simulink model "KinematicModelG"  (R2016b)
settings: Solver=ode45  StartTime=0.0  StopTime=2  RelTol=1e-3
settings Model: Creator=Daslab  LastModifiedBy=Daslab
settings SolverCC: ShapePreserveControl=EnableAll

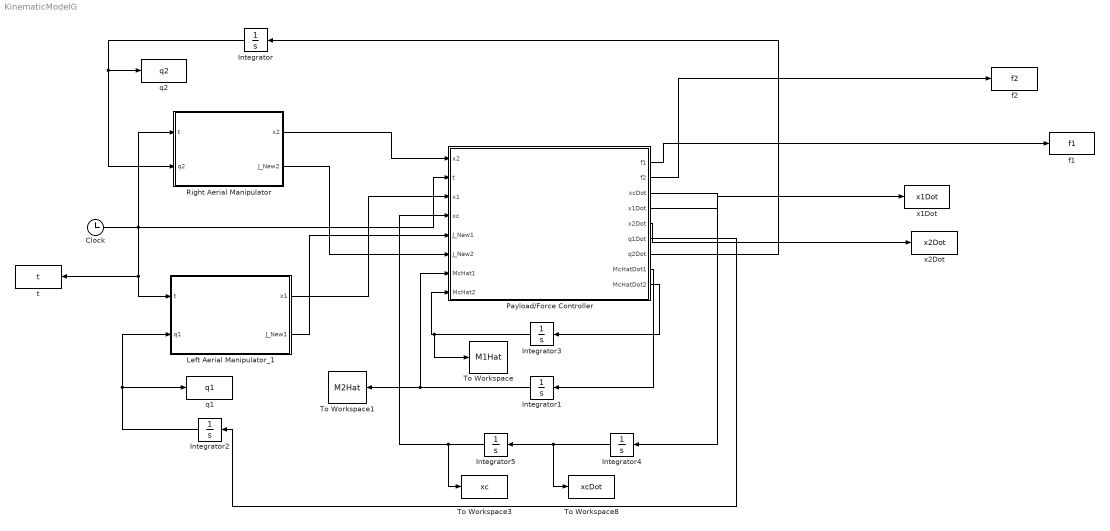
== system KinematicModelG ==
  Clock : Clock
  Integrator : Integrator  InitialCondition=[0.0;0.35;0.68;0;0;0.1;0;pi/2];
  Integrator1 : Integrator
  Integrator2 : Integrator  InitialCondition=[0.1;-0.35;0.7;0;0;-0.1;0;-pi/2];
  Integrator3 : Integrator
  Integrator4 : Integrator  InitialCondition=[0;0;0]
  Integrator5 : Integrator  InitialCondition=[0;0;0.5]
  Left Aerial Manipulator_1 : MATLAB Function  TreatAsAtomicUnit=on
  Payload/Force Controller : MATLAB Function  TreatAsAtomicUnit=on
  Right Aerial Manipulator : MATLAB Function  TreatAsAtomicUnit=on
  To Workspace : ToWorkspace  VariableName=M1Hat  SampleTime=-1
      settings: Save2DSignal=2-D array (concatenate along first dimension)
  To Workspace1 : ToWorkspace  VariableName=M2Hat  SampleTime=-1
      settings: Save2DSignal=2-D array (concatenate along first dimension)
  To Workspace3 : ToWorkspace  VariableName=xc  SampleTime=-1
  To Workspace8 : ToWorkspace  VariableName=xcDot  SampleTime=-1
  f1 : ToWorkspace  VariableName=f1  SampleTime=-1
  "f2 " : ToWorkspace  VariableName=f2  SampleTime=-1
  q1 : ToWorkspace  VariableName=q1  SampleTime=-1
  q2 : ToWorkspace  VariableName=q2  SampleTime=-1
  t : ToWorkspace  VariableName=t  SampleTime=-1
  x1Dot : ToWorkspace  VariableName=x1Dot  SampleTime=-1
  x2Dot : ToWorkspace  VariableName=x2Dot  SampleTime=-1
  wires:
  Integrator/1 -> q2/1, Right Aerial Manipulator/2(q2)
  Clock/1 -> t/1, Left Aerial Manipulator_1/1(t), Right Aerial Manipulator/1(t), Payload/Force Controller/2(t)
  Left Aerial Manipulator_1/1(x1) -> Payload/Force Controller/3(x1)
  Right Aerial Manipulator/1(x2) -> Payload/Force Controller/1(x2)
  Integrator4/1 -> To Workspace8/1, Integrator5/1
  Payload/Force Controller/3(xcDot) -> Integrator4/1
  Integrator5/1 -> To Workspace3/1, Payload/Force Controller/4(xc)
  Payload/Force Controller/1(f1) -> f1/1
  Payload/Force Controller/2(f2) -> "f2 "/1
  Payload/Force Controller/6(q1Dot) -> Integrator2/1
  Integrator2/1 -> q1/1, Left Aerial Manipulator_1/2(q1)
  Payload/Force Controller/5(x2Dot) -> x2Dot/1
  Payload/Force Controller/4(x1Dot) -> x1Dot/1
  Payload/Force Controller/7(q2Dot) -> Integrator/1
  Right Aerial Manipulator/2(J_New2) -> Payload/Force Controller/6(J_New2)
  Left Aerial Manipulator_1/2(J_New1) -> Payload/Force Controller/5(J_New1)
  Payload/Force Controller/9(McHatDot2) -> Integrator3/1
  Integrator3/1 -> To Workspace/1, Payload/Force Controller/8(McHat2)
  Payload/Force Controller/8(McHatDot1) -> Integrator1/1
  Integrator1/1 -> To Workspace1/1, Payload/Force Controller/7(McHat1)

== matlab function KinematicModelG/Left Aerial Manipulator_1 ==
  data: t input; x1 output; q1 input; J_New1 output
function [x1,J_New1] = LeftAerialManipulator(t,q1)
%Kinematics of Left Aerial Manipulator
xb1 = q1(1); 
yb1 = q1(2);
zb1 = q1(3);
psi1 = q1(4);      % z angle in the order ZYX [psi1 theta1 phi1] -->> [Zangle Yangle Xangle]
theta1 = q1(5);    % y angle
phi1 = q1(6);      % x angle 
n11 = q1(7); 
n21 = q1(8);

x_dot1 = 0.2;
y_dot1 = 0.2;
z_dot1 = 0;
phi_dot1 = 0.02;  % x angle 
theta_dot1 = 0;   % y anlge 
psi_dot1 = 0;     % z angle  in the order ZYX  [psiDot thetaDot phiDot] -->> [z y x]Dot
n1_dot1 = 0;
n2_dot1 = 0;

mUAV = 5.0; 
mLink1 = 0.5; 
mLink2 = 0.5;
l1 = 0.2; 
l2 = 0.2;
 
m1 = mUAV + mLink1 + mLink2; 

% Rotation matrix
R_b1 = [ cos(psi1)*cos(theta1), cos(psi1)*sin(phi1)*sin(theta1) - cos(phi1)*sin(psi1), sin(phi1)*sin(psi1) + cos(phi1)*cos(psi1)*sin(theta1); 
      cos(theta1)*sin(psi1), cos(phi1)*cos(psi1) + sin(phi1)*sin(psi1)*sin(theta1),   cos(phi1)*sin(psi1)*sin(theta1) - cos(psi1)*sin(phi1);
      -sin(theta1),         cos(theta1)*sin(phi1),                              cos(phi1)*cos(theta1)];

  
T_b1 = [ 0, -sin(psi1), cos(psi1)*cos(theta1); 
        0,  cos(psi1), cos(theta1)*sin(psi1); 
        1,         0,         -sin(theta1)];

% Forward Kinematics
p_b = [xb1 yb1 zb1]'; %postion of UAV with respect to inertial frame
p_b_dot1 = [x_dot1 y_dot1 z_dot1]';
n_dot1 = [n1_dot1 n2_dot1]'; % joint angles rate 
h1 = [1 0 0]'; 
P10 = [0 0 0.0]';
p1c = [0 0 -l1/2]';

R01 = expm((hat(h1))*n11);

p1c_b = P10 + R01*p1c;    % in base frame 
p1c_i = p_b + R_b1*p1c_b;  % in inertial frame

% position of center of link 2 
h2 = [0 1 0]';
p12 = [0 0 -l1]';
p2T = [0 l2 0]';
p2c = [0 l2/2 0]';

R12 = expm((hat(h2))*n21);
R02 = R01*R12;

% position of end effector 
p2_b1 = P10 + R01*p12 + R02*p2T; % in base frame
% disp(p2_b1);
% disp(x1);
% disp(y1);
% disp(z1);
x1 = p_b + R_b1*p2_b1;  % in inertial frame
% disp('x1'); 
% disp(x1);

% J2c = [h1 h2; hat(h1)*(R01*p12) hat(h2)*p2c_b];
% Jacobian for end effector 
JT1 = [h1 h2; hat(h1)*R01*p12 hat(h2)*p2_b1];
JwT1 = JT1(1:3,1:2);
JvT1 = JT1(4:6,1:2);



w_b1 = [phi_dot1*cos(psi1)*cos(theta1) - theta_dot1*sin(psi1); 
      theta_dot1*cos(psi1) + phi_dot1*cos(theta1)*sin(psi1);
                     psi_dot1 - phi_dot1*sin(theta1)];
                 
J_i1 = [eye(3,3),-hat(R_b1*p2_b1)*T_b1,R_b1*JvT1];
Ja1 = J_i1(:,1); 
Jb1 = J_i1(:,2);
Jd1 = J_i1(:,6);

J_New1 = [Ja1,Jb1,Jd1];

% q1Dot = inv(J_New1)*x1Dot;
% q1Dot = ones(3,1);
% x1Dot = p_b_dot1 + hat(w_b1)*R_b1*p2_b1 + R_b1*JvT1*n_dot1;    % end effector

== matlab function KinematicModelG/Right Aerial Manipulator ==
  data: x2 output; t input; q2 input; J_New2 output
function [x2,J_New2]   = RightAerialManipulator(t,q2)
% Agent 2 
% m2 = 1.0;
xb2 = q2(1); 
yb2 = q2(2);
zb2 = q2(3);
psi2 = q2(4); % z angle in the order ZYX - yaw pitch roll !!!
theta2 = q2(5);
phi2 = q2(6);
n12 = q2(7); 
n22 = q2(8);

x_dot2 = 0.2;
y_dot2 = 0.2;
z_dot2 = 0;
phi_dot2 = 0.02;
theta_dot2 = 0;
psi_dot2 = 0;
n1_dot1 = 0;
n2_dot1 = 0;

mUAV = 5.0; 
mLink1 = 0.5; 
mLink2 = 0.5;
l1 = 0.2; 
l2 = 0.2;
%  
m2 = mUAV + mLink1 + mLink2; 

% Rotation matrix
R_b2 = [ cos(psi2)*cos(theta2), cos(psi2)*sin(phi2)*sin(theta2) - cos(phi2)*sin(psi2), sin(phi2)*sin(psi2) + cos(phi2)*cos(psi2)*sin(theta2); 
      cos(theta2)*sin(psi2), cos(phi2)*cos(psi2) + sin(phi2)*sin(psi2)*sin(theta2),   cos(phi2)*sin(psi2)*sin(theta2) - cos(psi2)*sin(phi2);
      -sin(theta2),         cos(theta2)*sin(phi2),                              cos(phi2)*cos(theta2)];

% Transformation Matrix
T_b2 = [ 0, -sin(psi2), cos(psi2)*cos(theta2); 
        0,  cos(psi2), cos(theta2)*sin(psi2); 
        1,         0,         -sin(theta2)];
% Forward Kinematics
p_b2 = [xb2 yb2 zb2]'; %postion of UAV with respect to inertial frame
p_b_dot2 = [x_dot2 y_dot2 z_dot2]';
n_dot2 = [n1_dot1 n2_dot1]'; % joint angles rate 
h12 = [1 0 0]'; 
P102 = [0 0 0.0]';
p1c2 = [0 0 -l1/2]';

R012 = expm((hat(h12))*n12);

p1c_b2 = P102 + R012*p1c2;    % in base frame 
p1c_i2 = p_b2 + R_b2*p1c_b2;  % in inertial frame

% position of center of link 2 
h22 = [0 -1 0]';
p122 = [0 0 -l1]';
p2T2 = [0 -l2 0]';
p2c2 = [0 -l2/2 0]';

R122 = expm((hat(h22))*n22);
R022 = R012*R122;

% position of end effector 
p2_b2 = P102 + R012*p122 + R022*p2T2; % in base frame
% disp(p2_b1);
% disp(x1);
% disp(y1);
% disp(z1);
x2 = p_b2 + R_b2*p2_b2;  % in inertial frame
% disp('x2'); 
% disp(x2);


% J2c = [h1 h2; hat(h1)*(R01*p12) hat(h2)*p2c_b];
% Jacobian for end effector 
JT2 = [h12 h22; hat(h12)*R012*p122 hat(h22)*p2_b2];
JwT2 = JT2(1:3,1:2);
JvT2 = JT2(4:6,1:2);

w_b2 = [phi_dot2*cos(psi2)*cos(theta2) - theta_dot2*sin(psi2); 
      theta_dot2*cos(psi2) + phi_dot2*cos(theta2)*sin(psi2);
                     psi_dot2 - phi_dot2*sin(theta2)];
% x2Dot = p_b_dot2 + hat(w_b2)*R_b2*p2_b12 + R_b2*JvT12*n_dot2;    % end effector

J_i2 = [eye(3,3),-hat(R_b2*p2_b2)*T_b2,R_b2*JvT2];
Ja2 = J_i2(:,1); 
Jb2 = J_i2(:,2);
Jd2 = J_i2(:,6);   % phiDot to phi -->> X angle which is 6th variable in generalized coordinates

J_New2 = [Ja2,Jb2,Jd2];

% q2Dot = inv(J_New2)*x2Dot;
% q2Dot = ones(3,1);

== matlab function KinematicModelG/Payload//Force Controller ==
  data: f1 output; f2 output; xcDot output; x1Dot output; x2Dot output; x2 input; t input; x1 input; xc input; J_New1 input; q1Dot output; J_New2 input; q2Dot output; McHat1 input; McHat2 input; McHatDot1 output; McHatDot2 output
function [f1,f2,xcDot,x1Dot,x2Dot,q1Dot,q2Dot,McHatDot1,McHatDot2]  = PayLoad(x2,t,x1,xc,J_New1,J_New2,McHat1,McHat2)

%% Load 
Mc = 0.5; 
e = [0 0 1]';
g = 9.81;
% xc = [q(7);q(8);q(9)];
% xcDot = [q(10);q(11);q(12)];

theta = 0;
R_theta = [cos(theta) -sin(theta) 0;
           sin(theta) cos(theta)  0; 
           0          0           1];       
% xc = [0;0;0.5];
r1 = [0 -0.15 0]';
r2 = [0 0.15 0]';

a1 = xc + R_theta*r1; 

a2 = xc + R_theta*r2;

z1 = x1 - a1;
% z1
% max(z1)

z2 = x2 - a2;
k = 100;
f1 = k*z1; 
f2 = k*z2; 

% f1 = k*norm(z1)*z1;
% f2 = k*norm(z2)*z2;

% f_sg = 0.5*Mc*g + 10;
f1d = [0 2.0 McHat1*g]';
f2d = [0 -2.0 McHat2*g]';

v1d = [0.2 0 0]';
v2d = [0.2 0 0]';

% gamma = 30*eye(3,3);
% F1 = -gamma*(x1Dot - v1d) + f1d;
% F2 = -gamma*(x2Dot - v2d) + f2d; 
% 
% x1dDot = (F1 - f1)/m1; 
% x2dDot = (F2 - f2)/m2;
% f_z = [0 0 20]';
xcDot = (f1 + f2 - Mc*e*g)/Mc;
% 
% K1 = [.001 0 0;
%       0 .001 0;
%       0 0 .001];
K1 = 0.1;
K2 = K1;
x1Dot = K1*(f1d - f1) + v1d;
% x1Dot
x2Dot = K2*(f2d - f2) + v2d;
% x2Dot

McHatDot1 = -0.6*((x1Dot-v1d)'*g*e);
McHatDot2 = -0.4*((x2Dot-v2d)'*g*e);

q1DotPrtl = inv(J_New1)*x1Dot;
q1Dot = [q1DotPrtl(1),q1DotPrtl(2),0,0,0,q1DotPrtl(3),0,0]';

q2DotPrtl = inv(J_New2)*x2Dot;
q2Dot = [q2DotPrtl(1),q2DotPrtl(2),0,0,0,q2DotPrtl(3),0,0]';


% 
% J_i2 = [eye(3,3),-hat(R_b2*p2_b2)*T_b2,R_b2*JvT2];
% Ja2 = J_i2(:,1); 
% Jb2 = J_i2(:,2);
% Jd2 = J_i2(:,6);   % phiDot to phi -->> X angle which is 6th variable in generalized coordinates
% 
% J_New2 = [Ja2,Jb2,Jd2];
% 
% q2Dot = inv(J_New2)*x2Dot;
% 
% zDot(1:6,1)= [q1Dot;q2Dot];
% zDot(7:9,1)= q(10:12,1);
% zDot(10:12,1)= xcDot;
